simulink model "Validation_test_model_2016"  (Simulink 8.5)
settings: Solver=FixedStepDiscrete  StartTime=0.0  StopTime=10.0  RelTol=1e-3
PreLoadFcn:
  | try, eval([bdroot '_setup']); catch, eval('model_setup', ''); end
InitFcn:
  | try, eval([bdroot '_setup']); catch, eval('model_setup', ''); end
undefined symbols (not defined in the file): a, b, c, d, e, ECU565, f, motohawk_build_version, motohawk_trunc_name, motohawk_vardec_path, sigbuilder_block
libraries: MotoHawk_lib x32, motohawk_annotations_lib x6
Description:
  | Template_of_Final_project
CloseFcn:
  | try, eval([bdroot '_close']); catch, eval('model_close', ''); end
settings Model: MotoHawkBuildVersion=005  MotoHawkBuildStats=struct('TotalFLASH',{0},'TotalEEPROM',{0},'TotalRAM',{0},'AppFLASH',{0},'AppEEPROM',{0},'AppRAM',{0},'HeapRAM',{0},'BuildSuccessCount',{5},'BuildErrorCount',{0})  MotoHawkModelSavedName=Validation_test_model_2016  MotoHawkModelGUID=C2EF9B66-05E6-4C78-8577-5B0F5D47F813  MotoHawkModelOpenTime=2016 3 30 18 59 53.069  MotoHawkModelElapsedTime=96188.182  MotoHawkBuildInfo=struct('model_name',{'Model_in_Template'},'motohawk_version',{'2010a_sp1.49'},'motohawk_component_version',{'0.0.7'},'matlab_version',{'7.10.0'},'build_version',{'004'},'module_type',{'ECU565-128'},'layout_type',{'DEV'},'processor_family',{'PPC'},'processor_type',{'MPC565'},'toolchain_vendor',{'gcc-powerpc-eabi'},'toolchain_version',{'4.4.0'},'component',{0},'archive_file',{'PCM128.a'},'enable_build',{1},'fptype',{0},'flash_size',{1048576},'ee_size',{8192},'ram_size',{36864},'decram_size',{4096},'module_memory_def',{'MPC565_ModMemoryDef_Dev'},'eri_table0_rev',{9},'max_eri_table_size',{65535},'use_debug_vardecs',{1},'use_info_vardecs',{1},'fgnd_base_period_ms',{5},'bgnd_base_period_ms',{50},'root_build_dir',{'C:\MEEM_5750_Final_Project\LeiFeng'},'build_dir',{'C:\MEEM_5750_Final_Project\LeiFeng\Model_in_Template_Build'},'dll_name',{'Model_in__004'},'srz_name',{'Model_in_Template_004'},'fgnd_stack_size',{3072},'fgnd_angle_stack_size',{0},'bgnd_stack_size',{2048},'idle_stack_size',{1024},'irq_stack_size',{1536},'heap_size',{4096},'heap_margin',{409},'install_dll_dir',{'C:\ECUFiles\TDBDLL\'},'install_srz_dir',{'C:\ECUFiles\Programs'},'app_int_stack_size',{1024},'shutdown_stack_size',{1024},'mingw_dir',{'C:\PROGRA~1\Woodward\DEVELO~1\TOOLCH~1\GCC\win32-pe\4_4_0\'},'motohawk_dir',{'C:\PROGRA~1\Woodward\MCS\MotoHawk\2010A_~1.49'},'toolchain_dir',{'C:\Program Files\Woodward\DevelopmentTools\Toolchains\GCC\powerpc-eabi\4_4_0\'},'matlab_root',{'C:\Program Files\matlab2010a'},'model_guid',{'02501405-a1e3-47c9-ad-9c-d2-3e-71-52-84'},'build_guid',{'964a0459-529b-4d6f-81-45-cd-35-ed-ff-d3'},'token_guid',{'FDBF7FB80457F546A307B1464AF6A8B8'})  MotoHawkBuildGUID=964a0459-529b-4d6f-81-45-cd-35-ed-ff-d3  MotoHawkBuildDirectory=C:\Users\Piyush\Desktop\des proj\Validation_test_model_2016_Build  Creator=weiluo  LastModifiedBy=Piyush
settings ConfigSet: Description="This Simulink Configuration Set is preconfigured  for the MotoHawk target \"ECU565-128\"."
settings DataIOCC: SignalLoggingSaveFormat=Dataset
settings OptimizationCC: InlineParams=on  InlineInvariantSignals=on  EnhancedBackFolding=on  ExpressionDepthLimit=128  InitFltsAndDblsToZero=on  NoFixptDivByZeroProtection=on  EfficientFloat2IntCast=on  OptimizeModelRefInitCode=on  LifeSpan=1
settings DebuggingCC: InheritedTsInSrcMsg=none  TasksWithSamePriorityMsg=none  FcnCallInpInsideContextMsg=EnableAllAsError  ModelReferenceIOMismatchMessage=warning  StateNameClashWarn=none
settings HardwareCC: ProdLargestAtomicInteger=Integer  ProdLargestAtomicFloat=Float  ProdEndianess=BigEndian  ProdHWDeviceType=Specified
settings ModelReferenceCC: UpdateModelReferenceTargets=IfOutOfDate  CheckModelReferenceTargetMessage=warning  ModelReferenceNumInstancesAllowed=Single
settings RTWCC: SystemTargetFile=motohawk_ert_rtw.tlc  MakeCommand=make_rtw_motohawk  TemplateMakefile=motohawk_ert_rtw.tmf  Description=MotoHawk(tm) Rapid Prototyping
settings CodeAppCC: IgnoreCustomStorageClasses=off  MaxIdLength=100  CustomSymbolStrType=$N$R$M  CustomSymbolStrField=$H$N$M  InternalIdentifier=Classic
settings STFCustomTargetCC: ERTMultiwordTypeDef=User defined  ERTMultiwordLength=0  IncludeMdlTerminateFcn=off  GeneratePreprocessorConditionals=Disable all  CombineOutputUpdateFcns=on  SuppressErrorStatus=on  ERTCustomFileBanners=on  SupportContinuousTime=off  SupportNonInlinedSFcns=off  MATLABClassNameForMDSCustomization=Simulink.SoftwareTarget.ERTCustomization  GRTInterface=off  SystemTargetFile=motohawk_ert_rtw.tlc
settings ERTTargetCC: ERTMultiwordTypeDef=User defined  ERTMultiwordLength=0  MultiwordLength=2048  ParMdlRefBuildCompliant=off  CompOptLevelCompliant=off  ConcurrentExecutionCompliant=off  IncludeMdlTerminateFcn=off  GeneratePreprocessorConditionals=Disable all  SuppressErrorStatus=on  ERTFirstTimeCompliant=off  ModelStepFunctionPrototypeControlCompliant=off  CPPClassGenCompliant=off  InlinedParameterPlacement=NonHierarchical  ERTCustomFileTemplate=motohawk_file_process.tlc  ConvertIfToSwitch=off  SuppressUnreachableDefaultCases=off
settings CustomProperty: DataType=string  Value=ECU565-128

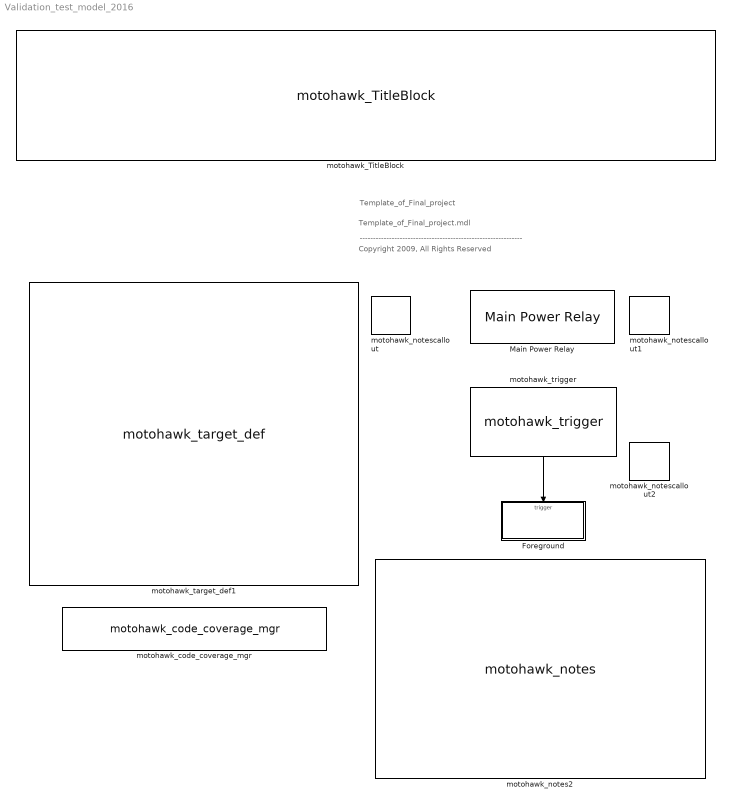
== system Validation_test_model_2016 ==
  note: Template_of_Final_project
  note: Template_of_Final_project.mdl
  note: -------------------------------------------------------------
  note: Copyright 2009, All Rights Reserved
  Foreground : Subsystem  TreatAsAtomicUnit=on
      mask init:
      | SampleTime = 0.005;
      | lbl = sprintf('%d ms', SampleTime * 1000);
      settings: RTWSystemCode=Nonreusable function  RTWFcnNameOpts=Use subsystem name  RTWFileNameOpts=Use function name
      mask Display: disp(lbl);
  Main Power Relay : MotoHawk_lib/Extra Development Blocks/Main Power Relay  on_delay_count=2  off_delay_count=5  ecup_threshold=100  group='System | Main Power Relay'
  motohawk_TitleBlock : motohawk_annotations_lib/motohawk_TitleBlock  BlockType_='Mototron_Title_Block'  ttl="[  strrep(get_param(bdroot, 'Description') , '_', '\\_')  '\\newline\\rm'  'Top-level root of model:  '   strrep(bdroot, '_', '\\_') '.mdl'  ]"  copyright="'THE INFORMATION CONTAINED IN THIS\\newlineDRAWING IS THE SOLE PROPERTY OF\\newlineWOODWARD.  ANY REPRODUCTION IN\\newline PART OR AS A WHOLE WITHOUT THE\\newlineWRITTEN PERMISSION OF WOODWARD\\newline IS PROHIBITED.\\fontsize{16}\\rm\\copyright\\rm\\fontsize{10} 2009'"  address='\fontsize{22}\it\fontname{Arial Black}Woodward \fontname{Arial}\fontsize{10}\newline1000 East Drake Road, Fort Collins, CO, 80525\newlinemcs.woodward.com (866) 588-0494'  image_file='mh.jpg'  pretty_print=on  edit_text=|  edit_as=5
      | [
      | 
      | 
      | 
      | 
      | 
      | strrep(get_param(bdroot, 'Description') , '_', '\_')  '\newline\rm'
      | 
      | 
      | 
      | 
      | 
      | 'Top-level root of model:  '   strrep(bdroot, '_', '\_') '.mdl'
      | 
      | 
      | 
      | 
      | 
      | ]
  motohawk_code_coverage_mgr : MotoHawk_lib/Extra Development Blocks/motohawk_code_coverage_mgr  codegen=Always Generate Code Coverage Code  group='System | Code Coverage'
  motohawk_notes2 : motohawk_annotations_lib/motohawk_notes  BlockType_='Mototron_Notes'  desc="'\\fontname{wingdings 2}u\\fontname{arial}  The existence of a Target Definition block\\newlinesomewhere in the model sets it up as a\\newlineMotoHawk project, capable of being built to a\\newlineMotoTron target module.\\newline\\newline\\fontname{wingdings 2}v\\fontname{arial}  The Main Power Relay block monitors the\\newlinemodule power and controls the Main Power Relay\\newlineIt also performs startup and shutdown procedures\\newlinenecessary for EEPROM storage.  Most designs\\newlineshould contain this block\\newline\\newline\\fontname{wingdings 2}w\\fontname{arial}  All actions must be performed inside of a\\newlinefunction-call subsystem, triggered by a MotoHawk\\newlineentry-point trigger block, in order to be included in the\\newlinegenerated code.\\newline'"  edit_text=|  edit_as=2
      | \fontname{wingdings 2}u\fontname{arial}  The existence of a Target Definition block
      | 
      | 
      | somewhere in the model sets it up as a
      | 
      | 
      | MotoHawk project, capable of being built to a
      | 
      | 
      | Woodward target module.
      | 
      | 
      | 
      | 
      | 
      | \fontname{wingdings 2}v\fontname{arial}  The Main Power Relay block monitors the
      | 
      | 
      | module power and controls the Main Power Relay
      | 
      | 
      | It also performs startup and shutdown procedures
      | 
      | 
      | necessary for EEPROM storage.  Most designs
      | 
      | 
      | should contain this block
      | 
      | 
      | 
      | 
      | 
      | \fontname{wingdings 2}w\fontname{arial}  All actions must be performed inside of a
      | 
      | 
      | function-call subsystem, triggered by a MotoHawk
      | 
      | 
      | entry-point trigger block, in order to be included in the
      | 
      | 
      | generated code.
  motohawk_notescallout : motohawk_annotations_lib/motohawk_notescallout  BlockType_='Mototron_NoteCall'  desc='\bf1'
  motohawk_notescallout1 : motohawk_annotations_lib/motohawk_notescallout  BlockType_='Mototron_NoteCall'  desc='\bf2'
  motohawk_notescallout2 : motohawk_annotations_lib/motohawk_notescallout  BlockType_='Mototron_NoteCall'  desc='\bf3'
  motohawk_target_def1 : MotoHawk_lib/motohawk_target_def  Priority=-65535  target=ECU565-128  layout=DEV  fptype=single (32 bits)  fgnd_stack_size=3*1024  fgnd_angle_stack_size=0  bgnd_stack_size=2*1024  idle_stack_size=1024  irq_stack_size=1536  app_int_stack_size=1024  shutdown_stack_size=1024  heap_size=4*1024  show_margins=off  fgnd_stack_margin=(3*1024) * 0.1  fgnd_angle_stack_margin=0  bgnd_stack_margin=(2*1024) * 0.1  idle_stack_margin=(1024) * 0.1  irq_stack_margin=(1536) * 0.1  app_int_stack_margin=(1024) * 0.1  shutdown_stack_margin=(1024) * 0.1  heap_margin=(4*1024) * 0.1  comp_name=bdroot  comp_img='KVASER_CAN_USB.jpg'  comp_security=No Encryption  comp_build_pass='mhbuild'  comp_sim_pass='mhsim'  comp_multi=off  show_filenames=off  dll_name=motohawk_trunc_name(bdroot, ['_' motohawk_build_version], 13)  srz_name=motohawk_trunc_name(bdroot, ['_' motohawk_build_version], 50)  build_dir='.'  comp_dir='.'
  motohawk_trigger : MotoHawk_lib/Trigger Blocks/motohawk_trigger  Tag=Trigger  Priority=0  trig_name=[]  trigger=FGND_RTI_PERIODIC  priority_order=0  inherited=off  run_disabled=off  override_app_monitor=off  target=ECU565_128
  wires:
  motohawk_trigger/1 -> Foreground/Trigger

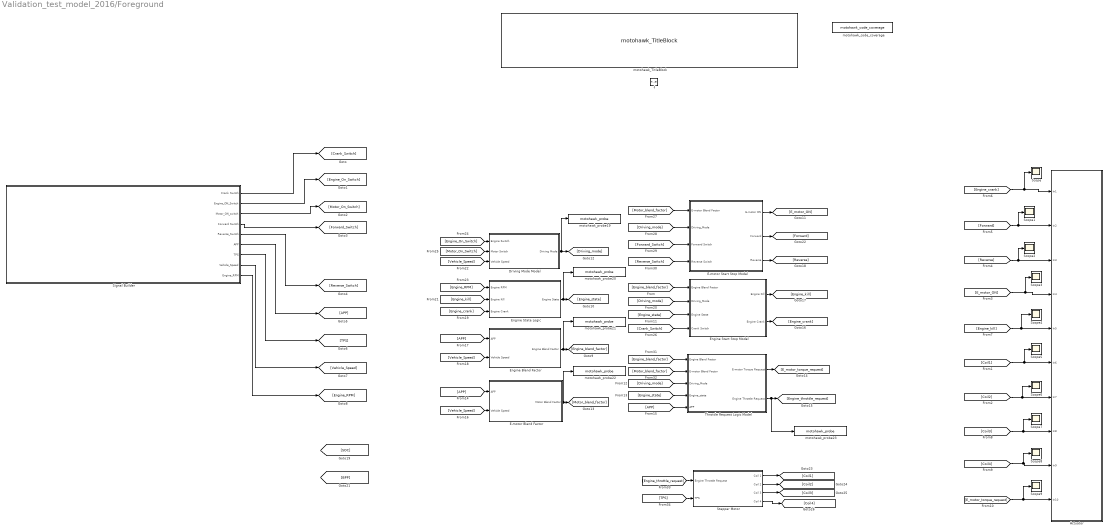
== system Validation_test_model_2016/Foreground ==
  f : TriggerPort  TriggerType=function-call
  Actuator : Subsystem
  Driving Mode Model : Subsystem
  E-motor Blend Factor : Subsystem
  E-motor Start Stop Model : Subsystem
  Engine Blend Factor : Subsystem
  Engine Start Stop Model : Subsystem
  Engine State Logic : Subsystem
  Scope{,1..9} (10 alike) : Scope
      Scope2 settings: TimeRange=10  SaveName=ScopeData2
      Scope3 settings: SaveName=ScopeData3
      Scope4 settings: SaveName=ScopeData4
      Scope5 settings: SaveName=ScopeData5
      Scope6 settings: SaveName=ScopeData6
      Scope7 settings: SaveName=ScopeData7
      Scope8 settings: SaveName=ScopeData8
      Scope9 settings: SaveName=ScopeData9
  Signal Builder : Subsystem  Tag=STV Subsys  LoadFcn=sigbuilder_block('load');  StartFcn=sigbuilder_block('start');  StopFcn=sigbuilder_block('stop');  ClipboardFcn=sigbuilder_block('clipboard');  mask(Sigbuilder block){}
      mask help: Simulink:masks:SigbuilderBlock_MD
      mask init:
      | if ~strcmp(get_param(bdroot(gcbh),'SimulationStatus'),'stopped') tuvar = sigbuilder_block('maskInit'); end
      settings: CopyFcn=sigbuilder_block('copy');  DeleteFcn=sigbuilder_block('delete');  ModelCloseFcn=sigbuilder_block('modelClose');  PreSaveFcn=sigbuilder_block('preSave');  PauseFcn=sigbuilder_block('pause');  ContinueFcn=sigbuilder_block('continue');  NameChangeFcn=sigbuilder_block('namechange');  OpenFcn=sigbuilder_block('open',[437.6 199.2 550.4 400 ]);  CloseFcn=sigbuilder_block('close');
      mask Display: plot(0, 0, 100, 100,[2, 2, 32, 32, 2], [68, 8, 8, 68, 68],[32, 2], [38, 38], [32, 19, 2],[53, 60, 44], [32, 17, 17, 2],[16, 16, 31, 31]);txt = getActiveGroup(gcbh);text(2, 100, txt,'verticalAlignment', 'top');
  Stepper Motor : Subsystem
  Throttle Request Logic Model : Subsystem
  motohawk_TitleBlock : motohawk_annotations_lib/motohawk_TitleBlock  BlockType_='Mototron_Title_Block'  ttl=[strrep(get_param(bdroot, 'Description') , '_', '\_') '\newline\rm' get_param(gcs, 'Name')]  copyright="'THE INFORMATION CONTAINED IN THIS\\newlineDRAWING IS THE SOLE PROPERTY OF\\newlineWOODWARD.  ANY REPRODUCTION IN\\newline PART OR AS A WHOLE WITHOUT THE\\newlineWRITTEN PERMISSION OF WOODWARD\\newline IS PROHIBITED.\\fontsize{16}\\rm\\copyright\\rm\\fontsize{10} 2009'"  address='\fontsize{22}\it\fontname{Arial Black}Woodward \fontname{Arial}\fontsize{10}\newline1000 East Drake Road, Fort Collins, CO, 80525\newlinemcs.woodward.com (866) 588-0494'  image_file='mh.jpg'  pretty_print=on  edit_text=[strrep(get_param(bdroot, 'Description') , '_', '\_') '\newline\rm' get_param(gcs, 'Name')]  edit_as=5
  motohawk_code_coverage : MotoHawk_lib/Extra Development Blocks/motohawk_code_coverage
  motohawk_probe19 : MotoHawk_lib/Calibration & Probing Blocks/motohawk_probe  nam='Driving_Mode'  show_more=off  name_source=Use Parameter  read_level=1  view_as=Number  enum_struct={'Disabled', 'Enabled'}  vector_style=Wide Row  use_help_units=off  help=''  units=''  use_header_enum=off  row_header_enum={}  col_header_enum={}  use_min_max=off  min_val=-inf  max_val=inf  use_precision=off  precision=''  gain=1  offset=0  exp=1  use_mototune_group=off  mototune_group=motohawk_vardec_path(gcb)
  motohawk_probe20 : MotoHawk_lib/Calibration & Probing Blocks/motohawk_probe  nam='Engine_State'  show_more=off  name_source=Use Parameter  read_level=1  view_as=Number  enum_struct={'Disabled', 'Enabled'}  vector_style=Wide Row  use_help_units=off  help=''  units=''  use_header_enum=off  row_header_enum={}  col_header_enum={}  use_min_max=off  min_val=-inf  max_val=inf  use_precision=off  precision=''  gain=1  offset=0  exp=1  use_mototune_group=off  mototune_group=motohawk_vardec_path(gcb)
  motohawk_probe21 : MotoHawk_lib/Calibration & Probing Blocks/motohawk_probe  nam='Engine_Blend_Factor'  show_more=off  name_source=Use Parameter  read_level=1  view_as=Number  enum_struct={'Disabled', 'Enabled'}  vector_style=Wide Row  use_help_units=off  help=''  units=''  use_header_enum=off  row_header_enum={}  col_header_enum={}  use_min_max=off  min_val=-inf  max_val=inf  use_precision=off  precision=''  gain=1  offset=0  exp=1  use_mototune_group=off  mototune_group=motohawk_vardec_path(gcb)
  motohawk_probe22 : MotoHawk_lib/Calibration & Probing Blocks/motohawk_probe  nam='Motor_blend_Factor'  show_more=off  name_source=Use Parameter  read_level=1  view_as=Number  enum_struct={'Disabled', 'Enabled'}  vector_style=Wide Row  use_help_units=off  help=''  units=''  use_header_enum=off  row_header_enum={}  col_header_enum={}  use_min_max=off  min_val=-inf  max_val=inf  use_precision=off  precision=''  gain=1  offset=0  exp=1  use_mototune_group=off  mototune_group=motohawk_vardec_path(gcb)
  motohawk_probe23 : MotoHawk_lib/Calibration & Probing Blocks/motohawk_probe  nam='Engine_Throttle_Request'  show_more=off  name_source=Use Parameter  read_level=1  view_as=Number  enum_struct={'Disabled', 'Enabled'}  vector_style=Wide Row  use_help_units=off  help=''  units=''  use_header_enum=off  row_header_enum={}  col_header_enum={}  use_min_max=off  min_val=-inf  max_val=inf  use_precision=off  precision=''  gain=1  offset=0  exp=1  use_mototune_group=off  mototune_group=motohawk_vardec_path(gcb)
  wires:
  [Forward] -> Scope1/1, Actuator/2(In2)
  [Reverse] -> Scope2/1, Actuator/3(In3)
  [E_motor_ON] -> Scope3/1, Actuator/4(In4)
  [Engine_kill] -> Scope4/1, Actuator/5(In5)
  [Coil1] -> Scope5/1, Actuator/6(In6)
  [Coil2] -> Scope6/1, Actuator/7(In7)
  [Coil3] -> Scope7/1, Actuator/8(In8)
  [Coil4] -> Scope8/1, Actuator/9(In9)
  [E_motor_torque_request] -> Scope9/1, Actuator/10(In10)
  [Engine_blend_factor] -> Engine Start Stop Model/1(Engine Blend Factor)
  Engine State Logic/1(Engine State) -> motohawk_probe20/1, [Engine_state]
  [Engine_state] -> Engine Start Stop Model/3(Engine State)
  Driving Mode Model/1(Driving Mode) -> motohawk_probe19/1, [Driving_mode]
  [Driving_mode] -> Engine Start Stop Model/2(Driving_Mode)
  [Crank_Switch] -> Engine Start Stop Model/4(Crank Switch)
  E-motor Blend Factor/1(Motor Blend Factor) -> motohawk_probe22/1, [Motor_blend_factor]
  [Motor_blend_factor] -> E-motor Start Stop Model/1(E-motor Blend Factor)
  [Driving_mode] -> E-motor Start Stop Model/2(Driving_Mode)
  [Forward_Switch] -> E-motor Start Stop Model/3(Forward Switch)
  [Reverse_Switch] -> E-motor Start Stop Model/4(Reverse Switch)
  [Engine_blend_factor] -> Throttle Request Logic Model/1(Engine Blend Factor)
  [Motor_blend_factor] -> Throttle Request Logic Model/2(E-motor Blend Factor)
  [Driving_mode] -> Throttle Request Logic Model/3(Driving_Mode)
  [Engine_state] -> Throttle Request Logic Model/4(Engine_state)
  [APP] -> E-motor Blend Factor/1(APP)
  [APP] -> Throttle Request Logic Model/5(APP)
  [Vehicle_Speed] -> E-motor Blend Factor/2(Vehicle Speed)
  [APP] -> Engine Blend Factor/1(APP)
  [Vehicle_Speed] -> Engine Blend Factor/2(Vehicle Speed)
  Throttle Request Logic Model/1(E-motor Torque Request) -> [E_motor_torque_request]
  Engine Start Stop Model/2(Engine Crank) -> [Engine_crank]
  Engine Start Stop Model/1(Engine Kill) -> [Engine_kill]
  E-motor Start Stop Model/3(Reverse) -> [Reverse]
  E-motor Start Stop Model/2(Forward) -> [Forward]
  E-motor Start Stop Model/1(E-motor ON) -> [E_motor_ON]
  [Engine_crank] -> Engine State Logic/3(Engine Crank)
  [Engine_kill] -> Engine State Logic/2(Engine Kill)
  [Engine_RPM] -> Engine State Logic/1(Engine RPM)
  [Vehicle_Speed] -> Driving Mode Model/3(Vehicle Speed)
  [Engine_On_Switch] -> Driving Mode Model/1(Engine Switch)
  [Motor_On_Switch] -> Driving Mode Model/2(Motor Switch)
  Engine Blend Factor/1(Engine Blend Factor) -> motohawk_probe21/1, [Engine_blend_factor]
  Throttle Request Logic Model/2(Engine Throttle Request) -> motohawk_probe23/1, [Engine_throttle_request]
  [Engine_throttle_request] -> Stepper Motor/1(Engine Throttle Request)
  [TPS] -> Stepper Motor/2(TPS)
  Stepper Motor/1(Coil 1) -> [Coil1]
  Stepper Motor/2(Coil 2) -> [Coil2]
  Stepper Motor/3(Coil 3) -> [Coil3]
  Stepper Motor/4(Coil 4) -> [Coil4]
  Signal Builder/1(Crank Switch) -> [Crank_Switch]
  Signal Builder/2(Engine_ON_Switch) -> [Engine_On_Switch]
  Signal Builder/3(Motor_ON_switch) -> [Motor_On_Switch]
  Signal Builder/4(Forward Switch) -> [Forward_Switch]
  Signal Builder/5(Reverse_Switch) -> [Reverse_Switch]
  Signal Builder/6(APP) -> [APP]
  [Engine_crank] -> Scope/1, Actuator/1(In1)
  Signal Builder/7(TPS) -> [TPS]
  Signal Builder/8(Vehicle_Speed) -> [Vehicle_Speed]
  Signal Builder/9(Engine_RPM) -> [Engine_RPM]

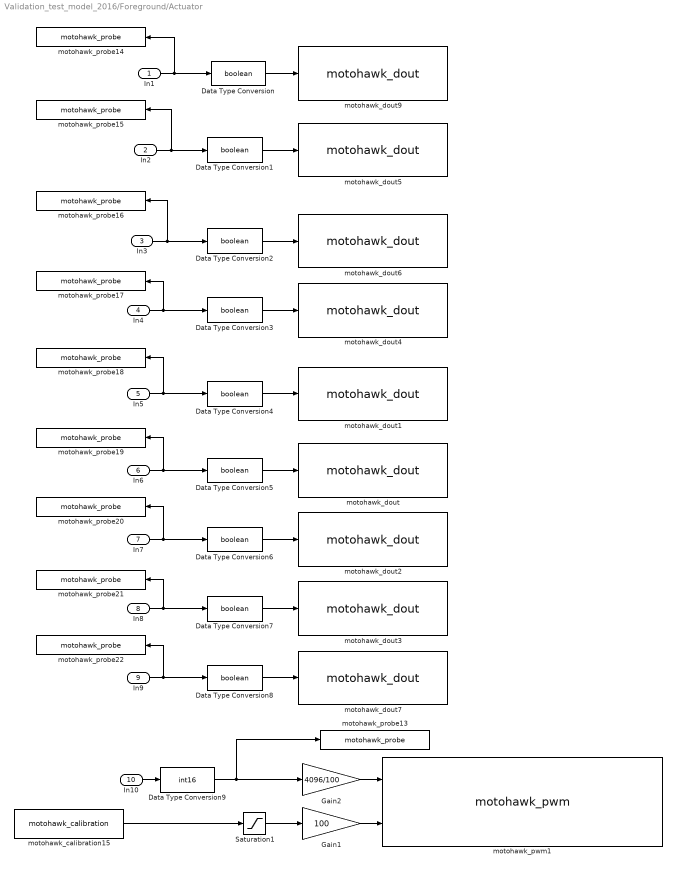
== system Validation_test_model_2016/Foreground/Actuator ==
  In1 : Inport
  In2 : Inport  Port=2
  In3 : Inport  Port=3
  In4 : Inport  Port=4
  In5 : Inport  Port=5
  In6 : Inport  Port=6
  In7 : Inport  Port=7
  In8 : Inport  Port=8
  In9 : Inport  Port=9
  In10 : Inport  Port=10
  Data Type Conversion{,1..8} (9 alike) : DataTypeConversion  OutDataTypeStr=boolean
  Data Type Conversion9 : DataTypeConversion  OutDataTypeStr=int16
  Gain1 : Gain  Gain=100  OutDataTypeStr=Inherit: Inherit via back propagation
  Gain2 : Gain  Gain=4096/100  OutDataTypeStr=Inherit: Inherit via back propagation
  Saturation1 : Saturate  UpperLimit=10000  LowerLimit=0
  motohawk_calibration15 : MotoHawk_lib/Calibration & Probing Blocks/motohawk_calibration  nam='Throttle_Frequency'  val=10000  storage=Calibration  show_more=on  name_source=Use Parameter  data_type=Inherit via back propagation  read_level=1  write_level=1  ovr_cals=on  view_as=Number  enum_struct={'Disabled', 'Enabled'}  vector_style=Wide Row  use_help_units=off  help=''  units=''  use_header_enum=off  row_header_enum={}  col_header_enum={}  use_min_max=off  min_val=-inf  max_val=inf  use_precision=off  precision=''  gain=1  offset=0  exp=1  use_mototune_group=off  mototune_group=motohawk_vardec_path(gcb)  data_stores=motohawk_sfun_calibration_data_stores
  motohawk_dout : MotoHawk_lib/Digital I//O Blocks/motohawk_dout  resource_name=[]  text_resource=LSD5  target=ECU565-128  use_diag=off  use_vardec=off  nam='DOUT'  read_level=1  write_level=1  group='System | I/O Pins | Outputs Config'
  motohawk_dout1 : MotoHawk_lib/Digital I//O Blocks/motohawk_dout  resource_name=[]  text_resource=LSD9  target=ECU565-128  use_diag=off  use_vardec=off  nam='DOUT'  read_level=1  write_level=1  group='System | I/O Pins | Outputs Config'
  motohawk_dout2 : MotoHawk_lib/Digital I//O Blocks/motohawk_dout  resource_name=[]  text_resource=LSD6  target=ECU565-128  use_diag=off  use_vardec=off  nam='DOUT'  read_level=1  write_level=1  group='System | I/O Pins | Outputs Config'
  motohawk_dout3 : MotoHawk_lib/Digital I//O Blocks/motohawk_dout  resource_name=[]  text_resource=LSD7  target=ECU565-128  use_diag=off  use_vardec=off  nam='DOUT'  read_level=1  write_level=1  group='System | I/O Pins | Outputs Config'
  motohawk_dout4 : MotoHawk_lib/Digital I//O Blocks/motohawk_dout  resource_name=[]  text_resource=LSD4  target=ECU565-128  use_diag=off  use_vardec=off  nam='DOUT'  read_level=1  write_level=1  group='System | I/O Pins | Outputs Config'
  motohawk_dout5 : MotoHawk_lib/Digital I//O Blocks/motohawk_dout  resource_name=[]  text_resource=LSD2  target=ECU565-128  use_diag=off  use_vardec=off  nam='DOUT'  read_level=1  write_level=1  group='System | I/O Pins | Outputs Config'
  motohawk_dout6 : MotoHawk_lib/Digital I//O Blocks/motohawk_dout  resource_name=[]  text_resource=LSD3  target=ECU565-128  use_diag=off  use_vardec=off  nam='DOUT'  read_level=1  write_level=1  group='System | I/O Pins | Outputs Config'
  motohawk_dout7 : MotoHawk_lib/Digital I//O Blocks/motohawk_dout  resource_name=[]  text_resource=LSD8  target=ECU565-128  use_diag=off  use_vardec=off  nam='DOUT'  read_level=1  write_level=1  group='System | I/O Pins | Outputs Config'
  motohawk_dout9 : MotoHawk_lib/Digital I//O Blocks/motohawk_dout  resource_name=[]  text_resource=LSD1  target=ECU565-128  use_diag=off  use_vardec=off  nam='DOUT'  read_level=1  write_level=1  group='System | I/O Pins | Outputs Config'
  motohawk_probe13 : MotoHawk_lib/Calibration & Probing Blocks/motohawk_probe  nam='Emotor_Throttle_Request'  show_more=off  name_source=Use Parameter  read_level=1  view_as=Number  enum_struct={'Disabled', 'Enabled'}  vector_style=Wide Row  use_help_units=off  help=''  units=''  use_header_enum=off  row_header_enum={}  col_header_enum={}  use_min_max=off  min_val=-inf  max_val=inf  use_precision=off  precision=''  gain=1  offset=0  exp=1  use_mototune_group=off  mototune_group=motohawk_vardec_path(gcb)
  motohawk_probe14 : MotoHawk_lib/Calibration & Probing Blocks/motohawk_probe  nam='Engine_Crank'  show_more=off  name_source=Use Parameter  read_level=1  view_as=Number  enum_struct={'Disabled', 'Enabled'}  vector_style=Wide Row  use_help_units=off  help=''  units=''  use_header_enum=off  row_header_enum={}  col_header_enum={}  use_min_max=off  min_val=-inf  max_val=inf  use_precision=off  precision=''  gain=1  offset=0  exp=1  use_mototune_group=off  mototune_group=motohawk_vardec_path(gcb)
  motohawk_probe15 : MotoHawk_lib/Calibration & Probing Blocks/motohawk_probe  nam='Foward'  show_more=off  name_source=Use Parameter  read_level=1  view_as=Number  enum_struct={'Disabled', 'Enabled'}  vector_style=Wide Row  use_help_units=off  help=''  units=''  use_header_enum=off  row_header_enum={}  col_header_enum={}  use_min_max=off  min_val=-inf  max_val=inf  use_precision=off  precision=''  gain=1  offset=0  exp=1  use_mototune_group=off  mototune_group=motohawk_vardec_path(gcb)
  motohawk_probe16 : MotoHawk_lib/Calibration & Probing Blocks/motohawk_probe  nam='Reverse'  show_more=off  name_source=Use Parameter  read_level=1  view_as=Number  enum_struct={'Disabled', 'Enabled'}  vector_style=Wide Row  use_help_units=off  help=''  units=''  use_header_enum=off  row_header_enum={}  col_header_enum={}  use_min_max=off  min_val=-inf  max_val=inf  use_precision=off  precision=''  gain=1  offset=0  exp=1  use_mototune_group=off  mototune_group=motohawk_vardec_path(gcb)
  motohawk_probe17 : MotoHawk_lib/Calibration & Probing Blocks/motohawk_probe  nam='E_Motor_On'  show_more=off  name_source=Use Parameter  read_level=1  view_as=Number  enum_struct={'Disabled', 'Enabled'}  vector_style=Wide Row  use_help_units=off  help=''  units=''  use_header_enum=off  row_header_enum={}  col_header_enum={}  use_min_max=off  min_val=-inf  max_val=inf  use_precision=off  precision=''  gain=1  offset=0  exp=1  use_mototune_group=off  mototune_group=motohawk_vardec_path(gcb)
  motohawk_probe18 : MotoHawk_lib/Calibration & Probing Blocks/motohawk_probe  nam='Engine_Kill'  show_more=off  name_source=Use Parameter  read_level=1  view_as=Number  enum_struct={'Disabled', 'Enabled'}  vector_style=Wide Row  use_help_units=off  help=''  units=''  use_header_enum=off  row_header_enum={}  col_header_enum={}  use_min_max=off  min_val=-inf  max_val=inf  use_precision=off  precision=''  gain=1  offset=0  exp=1  use_mototune_group=off  mototune_group=motohawk_vardec_path(gcb)
  motohawk_probe19 : MotoHawk_lib/Calibration & Probing Blocks/motohawk_probe  nam='Coil_1'  show_more=off  name_source=Use Parameter  read_level=1  view_as=Number  enum_struct={'Disabled', 'Enabled'}  vector_style=Wide Row  use_help_units=off  help=''  units=''  use_header_enum=off  row_header_enum={}  col_header_enum={}  use_min_max=off  min_val=-inf  max_val=inf  use_precision=off  precision=''  gain=1  offset=0  exp=1  use_mototune_group=off  mototune_group=motohawk_vardec_path(gcb)
  motohawk_probe20 : MotoHawk_lib/Calibration & Probing Blocks/motohawk_probe  nam='Coil_2'  show_more=off  name_source=Use Parameter  read_level=1  view_as=Number  enum_struct={'Disabled', 'Enabled'}  vector_style=Wide Row  use_help_units=off  help=''  units=''  use_header_enum=off  row_header_enum={}  col_header_enum={}  use_min_max=off  min_val=-inf  max_val=inf  use_precision=off  precision=''  gain=1  offset=0  exp=1  use_mototune_group=off  mototune_group=motohawk_vardec_path(gcb)
  motohawk_probe21 : MotoHawk_lib/Calibration & Probing Blocks/motohawk_probe  nam='Coil_3'  show_more=off  name_source=Use Parameter  read_level=1  view_as=Number  enum_struct={'Disabled', 'Enabled'}  vector_style=Wide Row  use_help_units=off  help=''  units=''  use_header_enum=off  row_header_enum={}  col_header_enum={}  use_min_max=off  min_val=-inf  max_val=inf  use_precision=off  precision=''  gain=1  offset=0  exp=1  use_mototune_group=off  mototune_group=motohawk_vardec_path(gcb)
  motohawk_probe22 : MotoHawk_lib/Calibration & Probing Blocks/motohawk_probe  nam='Coil_4'  show_more=off  name_source=Use Parameter  read_level=1  view_as=Number  enum_struct={'Disabled', 'Enabled'}  vector_style=Wide Row  use_help_units=off  help=''  units=''  use_header_enum=off  row_header_enum={}  col_header_enum={}  use_min_max=off  min_val=-inf  max_val=inf  use_precision=off  precision=''  gain=1  offset=0  exp=1  use_mototune_group=off  mototune_group=motohawk_vardec_path(gcb)
  motohawk_pwm1 : MotoHawk_lib/Analog I//O Blocks/motohawk_pwm  res_name='Emotor_Throttle'  text_resource=EST 1  target=ECU565-128  freq_mode=-1  min_freq=2  use_max_freq=off  max_freq=42949672.96  use_enable=off  use_brake=off  output_current=off  output_fault_status=off  use_child=off  use_vardec=off  nam='PWM'  read_level=1  write_level=1  group='System | I/O Pins | Outputs Config'
  wires:
  Data Type Conversion9/1 -> motohawk_probe13/1, Gain2/1
  Data Type Conversion8/1 -> motohawk_dout7/1
  Data Type Conversion7/1 -> motohawk_dout3/1
  Data Type Conversion6/1 -> motohawk_dout2/1
  Data Type Conversion5/1 -> motohawk_dout/1
  Data Type Conversion4/1 -> motohawk_dout1/1
  Data Type Conversion3/1 -> motohawk_dout4/1
  Data Type Conversion2/1 -> motohawk_dout6/1
  Data Type Conversion1/1 -> motohawk_dout5/1
  Data Type Conversion/1 -> motohawk_dout9/1
  In9/1 -> Data Type Conversion8/1, motohawk_probe22/1
  In8/1 -> Data Type Conversion7/1, motohawk_probe21/1
  In7/1 -> Data Type Conversion6/1, motohawk_probe20/1
  In6/1 -> Data Type Conversion5/1, motohawk_probe19/1
  Saturation1/1 -> Gain1/1
  Gain2/1 -> motohawk_pwm1/1
  Gain1/1 -> motohawk_pwm1/2
  motohawk_calibration15/1 -> Saturation1/1
  In2/1 -> Data Type Conversion1/1, motohawk_probe15/1
  In5/1 -> Data Type Conversion4/1, motohawk_probe18/1
  In1/1 -> Data Type Conversion/1, motohawk_probe14/1
  In3/1 -> Data Type Conversion2/1, motohawk_probe16/1
  In4/1 -> Data Type Conversion3/1, motohawk_probe17/1
  In10/1 -> Data Type Conversion9/1

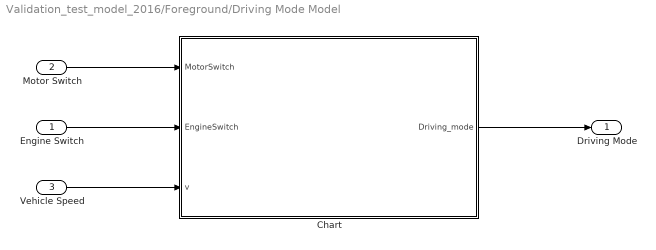
== system Validation_test_model_2016/Foreground/Driving Mode Model ==
  Engine Switch : Inport
  Motor Switch : Inport  Port=2
  Vehicle Speed : Inport  Port=3
  Chart : Stateflow chart  TreatAsAtomicUnit=on
  Driving Mode : Outport
  wires:
  Motor Switch/1 -> Chart/1(MotorSwitch)
  Engine Switch/1 -> Chart/2(EngineSwitch)
  Vehicle Speed/1 -> Chart/3(v)
  Chart/1(Driving_mode) -> Driving Mode/1

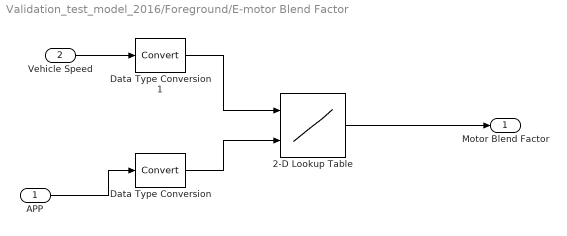
== system Validation_test_model_2016/Foreground/E-motor Blend Factor ==
  APP : Inport
  Vehicle Speed : Inport  Port=2
  2-D Lookup Table : Lookup_n-D  BreakpointsForDimension1=a  BreakpointsForDimension2=b  Table=c  InternalRulePriority=Speed  RndMeth=Simplest  InputSameDT=on
  Data Type Conversion : DataTypeConversion
  Data Type Conversion1 : DataTypeConversion
  Motor Blend Factor : Outport
  wires:
  Vehicle Speed/1 -> Data Type Conversion1/1
  APP/1 -> Data Type Conversion/1
  2-D Lookup Table/1 -> Motor Blend Factor/1
  Data Type Conversion/1 -> 2-D Lookup Table/2
  Data Type Conversion1/1 -> 2-D Lookup Table/1

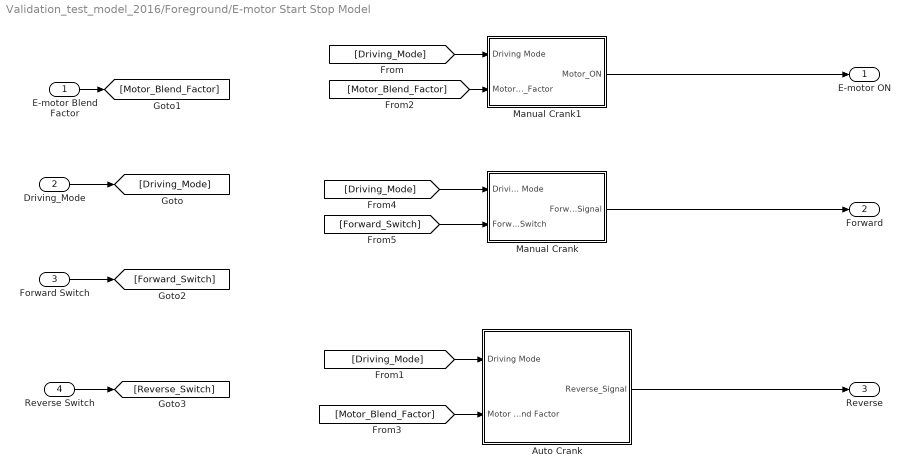
== system Validation_test_model_2016/Foreground/E-motor Start Stop Model ==
  E-motor Blend Factor : Inport
  Driving_Mode : Inport  Port=2
  Forward Switch : Inport  Port=3
  Reverse Switch : Inport  Port=4
  Auto Crank : Subsystem
  Manual Crank : Subsystem
  Manual Crank1 : Subsystem
  E-motor ON : Outport
  Forward : Outport  Port=2
  Reverse : Outport  Port=3
  wires:
  [Forward_Switch] -> Manual Crank/2(Forward Switch)
  Manual Crank1/1(Motor_ON) -> E-motor ON/1
  [Driving_Mode] -> Manual Crank1/1(Driving Mode)
  [Driving_Mode] -> Auto Crank/1(Driving Mode)
  [Motor_Blend_Factor] -> Manual Crank1/2(Motor_Blend_Factor)
  [Motor_Blend_Factor] -> Auto Crank/2(Motor Blend Factor)
  [Driving_Mode] -> Manual Crank/1(Driving Mode)
  E-motor Blend Factor/1 -> [Motor_Blend_Factor]
  Driving_Mode/1 -> [Driving_Mode]
  Forward Switch/1 -> [Forward_Switch]
  Reverse Switch/1 -> [Reverse_Switch]
  Auto Crank/1(Reverse_Signal) -> Reverse/1
  Manual Crank/1(Forward_Signal) -> Forward/1

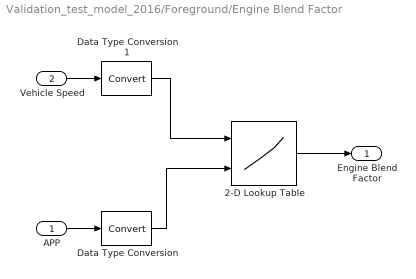
== system Validation_test_model_2016/Foreground/Engine Blend Factor ==
  APP : Inport
  Vehicle Speed : Inport  Port=2
  2-D Lookup Table : Lookup_n-D  BreakpointsForDimension1=d  BreakpointsForDimension2=e  Table=f  InternalRulePriority=Speed  RndMeth=Simplest  InputSameDT=on
  Data Type Conversion : DataTypeConversion
  Data Type Conversion1 : DataTypeConversion
  Engine Blend Factor : Outport
  wires:
  2-D Lookup Table/1 -> Engine Blend Factor/1
  APP/1 -> Data Type Conversion/1
  Vehicle Speed/1 -> Data Type Conversion1/1
  Data Type Conversion/1 -> 2-D Lookup Table/2
  Data Type Conversion1/1 -> 2-D Lookup Table/1

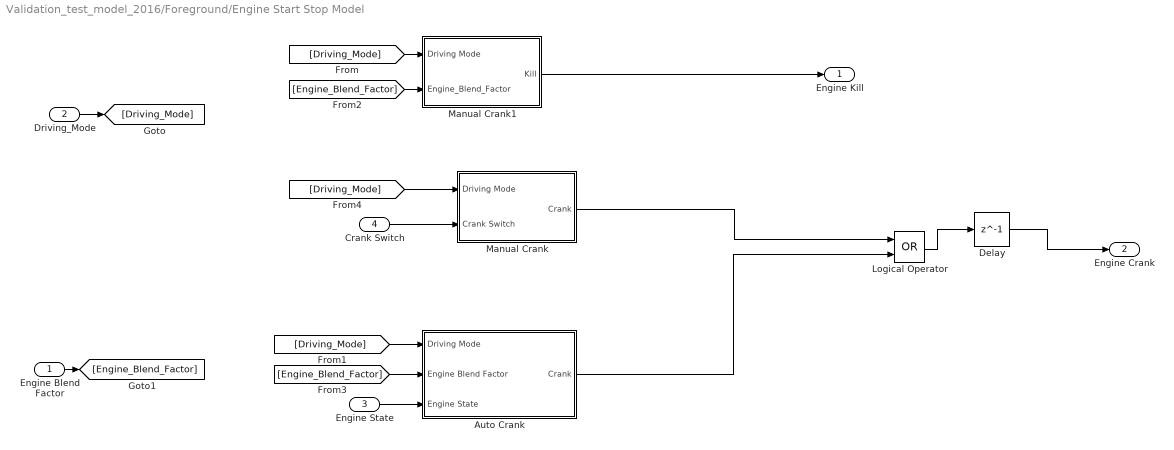
== system Validation_test_model_2016/Foreground/Engine Start Stop Model ==
  Engine Blend Factor : Inport
  Driving_Mode : Inport  Port=2
  Engine State : Inport  Port=3
  Crank Switch : Inport  Port=4
  Auto Crank : Subsystem
  Delay : Delay  DelayLength=1  InitialCondition=0
  Logical Operator : Logic  Operator=OR  AllPortsSameDT=off  OutDataTypeStr=boolean
  Manual Crank : Subsystem
  Manual Crank1 : Subsystem
  Engine Kill : Outport
  Engine Crank : Outport  Port=2
  wires:
  Logical Operator/1 -> Delay/1
  Crank Switch/1 -> Manual Crank/2(Crank Switch)
  Engine State/1 -> Auto Crank/3(Engine State)
  Manual Crank1/1(Kill) -> Engine Kill/1
  Driving_Mode/1 -> [Driving_Mode]
  Engine Blend Factor/1 -> [Engine_Blend_Factor]
  [Driving_Mode] -> Manual Crank1/1(Driving Mode)
  [Driving_Mode] -> Auto Crank/1(Driving Mode)
  [Engine_Blend_Factor] -> Manual Crank1/2(Engine_Blend_Factor)
  [Engine_Blend_Factor] -> Auto Crank/2(Engine Blend Factor)
  [Driving_Mode] -> Manual Crank/1(Driving Mode)
  Auto Crank/1(Crank) -> Logical Operator/2
  Manual Crank/1(Crank) -> Logical Operator/1
  Delay/1 -> Engine Crank/1

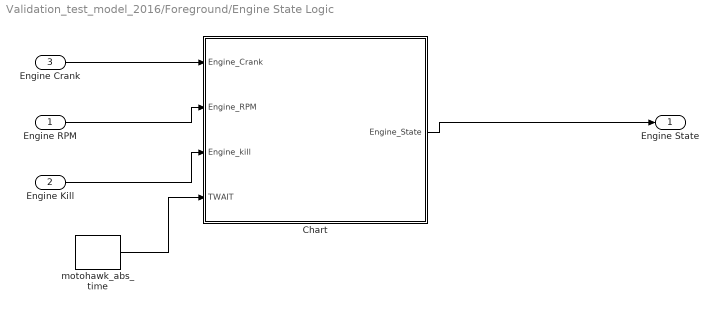
== system Validation_test_model_2016/Foreground/Engine State Logic ==
  Engine RPM : Inport
  Engine Kill : Inport  Port=2
  Engine Crank : Inport  Port=3
  Chart : Stateflow chart  TreatAsAtomicUnit=on
  motohawk_abs_time : MotoHawk_lib/Extra Development Blocks/motohawk_abs_time  mode=Seconds (double)  width=64 bit
  Engine State : Outport
  wires:
  Engine Crank/1 -> Chart/1(Engine_Crank)
  Engine Kill/1 -> Chart/3(Engine_kill)
  Engine RPM/1 -> Chart/2(Engine_RPM)
  Chart/1(Engine_State) -> Engine State/1
  motohawk_abs_time/1 -> Chart/4(TWAIT)

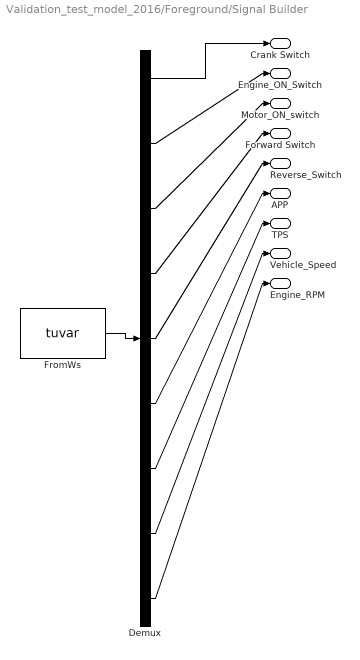
== system Validation_test_model_2016/Foreground/Signal Builder ==
  Demux : Demux  Tag=STV Demux  Outputs=9
  FromWs : FromWorkspace  Tag=STV FromWs  VariableName=tuvar  SigBuilderData=DataTag0  VnvData=DataTag1
      SigBuilderData=|
      | common.afterFinalStr = 'Extrapolate'
      | common.sampleTime = '-1'
      | dataSet.timeRange = [0 10]
      | dataSet.name = 'Group 1'
      | sbobj.Groups.Name = 'Group 1'
      | sbobj.Groups.Signals(1).Name = 'Crank Switch'
      | sbobj.Groups.Signals(1).XData = [0 4 6 10]
      | sbobj.Groups.Signals(1).YData = [0 0 0 0]
      | sbobj.Groups.Signals(2).Name = 'Engine_ON_Switch'
      | sbobj.Groups.Signals(2).XData = [0 10]
      | sbobj.Groups.Signals(2).YData = [1 1]
      | sbobj.Groups.Signals(3).Name = 'Motor_ON_switch'
      | sbobj.Groups.Signals(3).XData = [0 10]
      | sbobj.Groups.Signals(3).YData = [1 1]
      | sbobj.Groups.Signals(4).Name = 'Forward Switch'
      | sbobj.Groups.Signals(4).XData = [0 10]
      | sbobj.Groups.Signals(4).YData = [1 1]
      | sbobj.Groups.Signals(5).Name = 'Reverse_Switch'
      | sbobj.Groups.Signals(5).XData = [0 10]
      | sbobj.Groups.Signals(5).YData = [0 0.7]
      | sbobj.Groups.Signals(6).Name = 'APP'
      | sbobj.Groups.Signals(6).XData = [0 10]
      | sbobj.Groups.Signals(6).YData = [0 0.8]
      | sbobj.Groups.Signals(7).Name = 'TPS'
      | sbobj.Groups.Signals(7).XData = [0 1 10]
      | sbobj.Groups.Signals(7).YData = [0 2000 2000]
      | sbobj.Groups.Signals(8).Name = 'Vehicle_Speed'
      | sbobj.Groups.Signals(8).XData = [0 10]
      | sbobj.Groups.Signals(8).YData = [0 0]
      | sbobj.Groups.Signals(9).Name = 'Engine_RPM'
      | sbobj.Groups.Signals(9).XData = [0 10]
      | sbobj.Groups.Signals(9).YData = [0 0]
  Crank Switch : Outport  Tag=STV Outport
  Engine_ON_Switch : Outport  Tag=STV Outport  Port=2
  Motor_ON_switch : Outport  Tag=STV Outport  Port=3
  Forward Switch : Outport  Tag=STV Outport  Port=4
  Reverse_Switch : Outport  Tag=STV Outport  Port=5
  APP : Outport  Tag=STV Outport  Port=6
  TPS : Outport  Tag=STV Outport  Port=7
  Vehicle_Speed : Outport  Tag=STV Outport  Port=8
  Engine_RPM : Outport  Tag=STV Outport  Port=9
  wires:
  Demux/1 -> Crank Switch/1
  FromWs/1 -> Demux/1
  Demux/2 -> Engine_ON_Switch/1
  Demux/3 -> Motor_ON_switch/1
  Demux/4 -> Forward Switch/1
  Demux/5 -> Reverse_Switch/1
  Demux/6 -> APP/1
  Demux/7 -> TPS/1
  Demux/8 -> Vehicle_Speed/1
  Demux/9 -> Engine_RPM/1

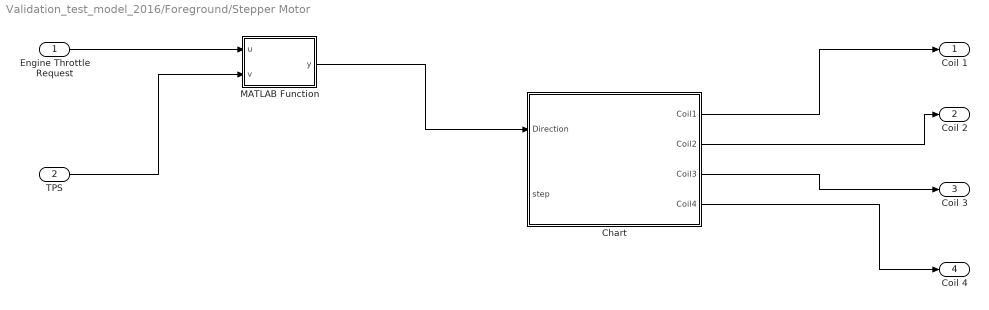
== system Validation_test_model_2016/Foreground/Stepper Motor ==
  Engine Throttle Request : Inport
  TPS : Inport  Port=2
  Chart : Stateflow chart  TreatAsAtomicUnit=on
  MATLAB Function : MATLAB Function  TreatAsAtomicUnit=on
  Coil 1 : Outport
  Coil 2 : Outport  Port=2
  Coil 3 : Outport  Port=3
  Coil 4 : Outport  Port=4
  wires:
  Engine Throttle Request/1 -> MATLAB Function/1(u)
  TPS/1 -> MATLAB Function/2(v)
  MATLAB Function/1(y) -> Chart/1(Direction)
  Chart/1(Coil1) -> Coil 1/1
  Chart/2(Coil2) -> Coil 2/1
  Chart/3(Coil3) -> Coil 3/1
  Chart/4(Coil4) -> Coil 4/1

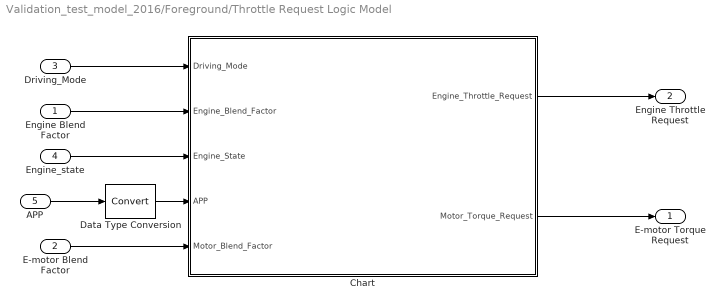
== system Validation_test_model_2016/Foreground/Throttle Request Logic Model ==
  Engine Blend Factor : Inport
  E-motor Blend Factor : Inport  Port=2
  Driving_Mode : Inport  Port=3
  Engine_state : Inport  Port=4
  APP : Inport  Port=5
  Chart : Stateflow chart  TreatAsAtomicUnit=on
  Data Type Conversion : DataTypeConversion
  E-motor Torque Request : Outport
  Engine Throttle Request : Outport  Port=2
  wires:
  Engine Blend Factor/1 -> Chart/2(Engine_Blend_Factor)
  E-motor Blend Factor/1 -> Chart/5(Motor_Blend_Factor)
  APP/1 -> Data Type Conversion/1
  Engine_state/1 -> Chart/3(Engine_State)
  Driving_Mode/1 -> Chart/1(Driving_Mode)
  Chart/2(Motor_Torque_Request) -> E-motor Torque Request/1
  Chart/1(Engine_Throttle_Request) -> Engine Throttle Request/1
  Data Type Conversion/1 -> Chart/4(APP)

== system Validation_test_model_2016/Foreground/E-motor Start Stop Model/Auto Crank ==
  Driving Mode : Inport
  Motor Blend Factor : Inport  Port=2
  Chart2 : Stateflow chart  TreatAsAtomicUnit=on
  Reverse_Signal : Outport
  wires:
  Chart2/1(Reverse) -> Reverse_Signal/1
  Driving Mode/1 -> Chart2/1(Driving_Mode)
  Motor Blend Factor/1 -> Chart2/2(Reverse_switch)

== system Validation_test_model_2016/Foreground/E-motor Start Stop Model/Manual Crank ==
  Driving Mode : Inport
  Forward Switch : Inport  Port=2
  Chart1 : Stateflow chart  TreatAsAtomicUnit=on
  Forward_Signal : Outport
  wires:
  Chart1/1(Forward) -> Forward_Signal/1
  Driving Mode/1 -> Chart1/1(Driving_Mode)
  Forward Switch/1 -> Chart1/2(Forward_switch)

== system Validation_test_model_2016/Foreground/E-motor Start Stop Model/Manual Crank1 ==
  Driving Mode : Inport
  Motor_Blend_Factor : Inport  Port=2
  Chart1 : Stateflow chart  TreatAsAtomicUnit=on
  Motor_ON : Outport
  wires:
  Driving Mode/1 -> Chart1/1(Driving_Mode)
  Motor_Blend_Factor/1 -> Chart1/2(Motor_Blend_Factor)
  Chart1/1(Motor_on) -> Motor_ON/1

== system Validation_test_model_2016/Foreground/Engine Start Stop Model/Auto Crank ==
  Driving Mode : Inport
  Engine Blend Factor : Inport  Port=2
  Engine State : Inport  Port=3
  Chart2 : Stateflow chart  TreatAsAtomicUnit=on
  Crank : Outport
  wires:
  Chart2/1(Automatic_crank) -> Crank/1
  Engine State/1 -> Chart2/3(Engine_State)
  Engine Blend Factor/1 -> Chart2/2(Engine_Blend_Factor)
  Driving Mode/1 -> Chart2/1(Driving_Mode)

== system Validation_test_model_2016/Foreground/Engine Start Stop Model/Manual Crank ==
  Driving Mode : Inport
  Crank Switch : Inport  Port=2
  Chart1 : Stateflow chart  TreatAsAtomicUnit=on
  Crank : Outport
  wires:
  Driving Mode/1 -> Chart1/1(Driving_Mode)
  Crank Switch/1 -> Chart1/2(Crank_Switch)
  Chart1/1(Manual_crank) -> Crank/1

== system Validation_test_model_2016/Foreground/Engine Start Stop Model/Manual Crank1 ==
  Driving Mode : Inport
  Engine_Blend_Factor : Inport  Port=2
  Chart1 : Stateflow chart  TreatAsAtomicUnit=on
  Kill : Outport
  wires:
  Engine_Blend_Factor/1 -> Chart1/2(Engine_Blend_Factor)
  Driving Mode/1 -> Chart1/1(Driving_Mode)
  Chart1/1(Engine_Kill) -> Kill/1

== stateflow chart Foreground/Engine State Logic/Chart ==
  state EngineCrank
    en: Time_stamp = TWAIT;
    during:Engine_State=2;
  state EngineOff
    during:Engine_State=1;
  state EngineStartFailSate
    during:Engine_State=5;
  state EngineOn
    en: Time_stamp = TWAIT;
    during:Engine_State=4;
  state EngineWarm_up
    en: Time_stamp = TWAIT;
    during: Engine_State=3;
  (default) -> EngineOff
  EngineOff -> EngineCrank : [Engine_Crank==1]
  EngineCrank -> EngineStartFailSate [order 2] : [Engine_RPM<=800&&TWAIT>Time_stamp+1]
  EngineCrank -> EngineWarm_up [order 1] : [Engine_RPM>800&&TWAIT>Time_stamp+0.6]
  EngineStartFailSate -> EngineOff
  EngineOn -> EngineOff : [Engine_RPM<50||Engine_kill==1]
  EngineWarm_up -> EngineStartFailSate [order 2] : [Engine_RPM<500 && TWAIT>Time_stamp+1]
  EngineWarm_up -> EngineOn [order 1] : [Engine_RPM>=500&&TWAIT>Time_stamp+1]
  data: Engine_Crank input double; Engine_RPM input double; Engine_kill input double; Engine_State output double; TWAIT input double; Time_stamp local double

== stateflow chart Foreground/E-motor Start Stop Model/Auto Crank/Chart2 ==
  state REVERSE_ON
    during: Reverse=1;
  state REVERSE_OFF
    during: Reverse=0;
  REVERSE_ON -> REVERSE_OFF : [Driving_Mode==2||Driving_Mode==3]
  REVERSE_OFF -> REVERSE_ON : [Driving_Mode==1&&Reverse_switch==1]
  (default) -> REVERSE_OFF
  data: Driving_Mode input double; Reverse_switch input double; Reverse output double

== stateflow chart Foreground/Driving Mode Model/Chart ==
  state Electric_solo_mode
    during:Driving_mode=1;
  state Blending_mode
    during:Driving_mode=2;
  state Engine_Solo_mode
    during: Driving_mode=3;
  (junction 41) -> Electric_solo_mode [order 2] : [MotorSwitch==1&&EngineSwitch==0&&v<1]
  Electric_solo_mode -> (junction 41) : [MotorSwitch==0&&v<1]
  (default) -> Blending_mode
  (junction 41) -> Blending_mode [order 3] : [EngineSwitch==0&&MotorSwitch==0&&v<1]
  Blending_mode -> (junction 41) : [EngineSwitch==0||MotorSwitch==0&&v<1]
  Engine_Solo_mode -> (junction 41) : [EngineSwitch==0&&v<1]
  (junction 41) -> Engine_Solo_mode [order 1] : [EngineSwitch==1&&MotorSwitch==0&&v<1]
  data: MotorSwitch input double; EngineSwitch input double; v input double; Driving_mode output double

== stateflow chart Foreground/Throttle Request Logic Model/Chart ==
  state BlendingMode
    state State1
      during: Engine_Throttle_Request=7.5;
      during:Motor_Torque_Request=APP*Motor_Blend_Factor;
    state State2
      during: Engine_Throttle_Request=(APP*Engine_Blend_Factor);
      during: Motor_Torque_Request=APP*Motor_Blend_Factor;
    State2 -> State1 : [Engine_State==2||Engine_State==3]
    State1 -> State2 : [Engine_State==1||Engine_State==4||Engine_State==5]
    (default) -> State2
  state ElectricSoloMode
    during: Engine_Throttle_Request=0;
    during: Motor_Torque_Request=APP;
  state EngineSoloMode
    during:Engine_Throttle_Request=APP;
    during: Motor_Torque_Request = 0;
  (default) -> ElectricSoloMode
  ElectricSoloMode -> (junction 66) : [Driving_Mode==2||Driving_Mode==3]
  (junction 66) -> ElectricSoloMode [order 1] : [Driving_Mode==1]
  (junction 66) -> BlendingMode [order 2] : [Driving_Mode==2]
  (junction 66) -> EngineSoloMode [order 3] : [Driving_Mode==3]
  BlendingMode -> (junction 66) : [Driving_Mode==2||Driving_Mode==1]
  EngineSoloMode -> (junction 66) : [Driving_Mode==2||Driving_Mode==1]
  data: Driving_Mode input double; Engine_Blend_Factor input double; Engine_State input double; APP input double; Motor_Blend_Factor input double; Engine_Throttle_Request output double; Motor_Torque_Request output double

== stateflow chart Foreground/E-motor Start Stop Model/Manual Crank/Chart1 ==
  state FORWARD_ON
    during: Forward=1;
  state FORWARD_OFF
    during: Forward=0;
  FORWARD_ON -> FORWARD_OFF : [Driving_Mode==3]
  FORWARD_OFF -> FORWARD_ON [order 1] : [Driving_Mode==2]
  FORWARD_OFF -> FORWARD_ON [order 2] : [Driving_Mode==1&&Forward_switch==1]
  (default) -> FORWARD_OFF
  data: Driving_Mode input double; Forward_switch input double; Forward output double

== stateflow chart Foreground/E-motor Start Stop Model/Manual Crank1/Chart1 ==
  state MOTOR_ON
    during: Motor_on=1;
  state MOTOR_OFF
    during: Motor_on=0;
  MOTOR_ON -> MOTOR_OFF [order 2] : [Driving_Mode==2&&Motor_Blend_Factor<0.01]
  MOTOR_ON -> MOTOR_OFF [order 1] : [Driving_Mode==3]
  MOTOR_OFF -> MOTOR_ON [order 1] : [Driving_Mode==1]
  MOTOR_OFF -> MOTOR_ON [order 2] : [Driving_Mode==2&&Motor_Blend_Factor>0.01]
  (default) -> MOTOR_OFF
  data: Driving_Mode input double; Motor_Blend_Factor input double; Motor_on output double

== matlab function Foreground/Stepper Motor/MATLAB Function ==
  data: u input double; y output double; v input double
function y= fcn(u,v)
%#codegen
Diff=u-v;
if abs(Diff)>1
    if Diff>0
        y=1;
    else y=0;
    end
else y=-1;
end

== stateflow chart Foreground/Engine Start Stop Model/Manual Crank/Chart1 ==
  state CRANK_ON
    during: Manual_crank=1;
  state CRANKOFF
    during: Manual_crank=0;
  CRANK_ON -> CRANKOFF : [Driving_Mode==1||Driving_Mode==2]
  CRANKOFF -> CRANK_ON : [Crank_Switch==1&&Driving_Mode==3]
  (default) -> CRANKOFF
  data: Driving_Mode input double; Crank_Switch input double; Manual_crank output double

== stateflow chart Foreground/Engine Start Stop Model/Auto Crank/Chart2 ==
  state CRANK_ON
    during: Automatic_crank=1;
  state CRANKOFF
    during: Automatic_crank=0;
  CRANK_ON -> CRANKOFF [order 1] : [Driving_Mode==1||Driving_Mode==3]
  CRANK_ON -> CRANKOFF [order 2] : [Driving_Mode==2&&Engine_Blend_Factor<0.01]
  CRANKOFF -> CRANK_ON : [Driving_Mode==2&&Engine_Blend_Factor>0.01&&Engine_State==1]
  (default) -> CRANKOFF
  data: Driving_Mode input double; Engine_Blend_Factor input double; Automatic_crank output double; Engine_State input double

== stateflow chart Foreground/Engine Start Stop Model/Manual Crank1/Chart1 ==
  state KILL_ON
    during: Engine_Kill=1;
  state KILL_OFF
    during: Engine_Kill=0;
  KILL_ON -> KILL_OFF [order 2] : [Driving_Mode==2&&Engine_Blend_Factor>0.01]
  KILL_ON -> KILL_OFF [order 1] : [Driving_Mode==3]
  KILL_OFF -> KILL_ON [order 1] : [Driving_Mode==1]
  KILL_OFF -> KILL_ON [order 2] : [Driving_Mode==2&&Engine_Blend_Factor<0.01]
  (default) -> KILL_OFF
  data: Driving_Mode input double; Engine_Blend_Factor input double; Engine_Kill output double

== stateflow chart Foreground/Stepper Motor/Chart ==
  state CW
    state step3
      during:
      Coil1=1;
      Coil2=0;
      Coil3=0;
      Coil4=1;
    state step1
      during:
      Coil1=1;
      Coil2=0;
      Coil3=1;
      Coil4=0;
    state step2
      during:
      Coil1=1;
      Coil2=0;
      Coil3=0;
      Coil4=0;
    state step6
      during:
      Coil1=0;
      Coil2=1;
      Coil3=0;
      Coil4=0;
    state step5
      during:
      Coil1=0;
      Coil2=1;
      Coil3=0;
      Coil4=1;
    state step4
      during:
      Coil1=0;
      Coil2=0;
      Coil3=0;
      Coil4=1;
    state step8
      during:
      Coil1=0;
      Coil2=0;
      Coil3=1;
      Coil4=0;
    state step7
      during:
      Coil1=0;
      Coil2=1;
      Coil3=1;
      Coil4=0;
    (default) -> CW.step1
    CW.step2 -> CW.step3 [order 2] : [step>2]
    CW.step1 -> CW.step2 : [step>1]
    CW.step3 -> CW.step2 [order 1] : [step<3]
    CW.step2 -> CW.step1 [order 1] : [step<2]
    CW.step3 -> CW.step4 [order 2] : [step>3]
    CW.step4 -> CW.step3 [order 1] : [step<4]
    CW.step4 -> CW.step5 [order 2] : [step>4]
    CW.step5 -> CW.step6 [order 2] : [step>5]
    CW.step6 -> CW.step5 [order 1] : [step<6]
    CW.step5 -> CW.step4 [order 1] : [step<5]
    CW.step6 -> CW.step7 [order 2] : [step>6]
    CW.step7 -> CW.step6 [order 1] : [step<7]
    CW.step7 -> CW.step8 [order 2] : [step>7]
    CW.step8 -> CW.step7 : [step<8]
  state CCW
    state step3
      during:
      Coil1=0;
      Coil2=1;
      Coil3=1;
      Coil4=0;
    state step1
      during:
      Coil1=1;
      Coil2=0;
      Coil3=1;
      Coil4=0;
    state step2
      during:
      Coil1=0;
      Coil2=0;
      Coil3=1;
      Coil4=0;
    state step6
      during:
      Coil1=0;
      Coil2=0;
      Coil3=0;
      Coil4=1;
    state step5
      during:
      Coil1=0;
      Coil2=1;
      Coil3=0;
      Coil4=1;
    state step4
      during:
      Coil1=0;
      Coil2=1;
      Coil3=0;
      Coil4=0;
    state step7
      during:
      Coil1=1;
      Coil2=0;
      Coil3=0;
      Coil4=1;
    state step8
      during:
      Coil1=1;
      Coil2=0;
      Coil3=0;
      Coil4=0;
    (default) -> CCW.step1
    CCW.step1 -> CCW.step2 : [step>1]
    CCW.step2 -> CCW.step3 [order 2] : [step>2]
    CCW.step3 -> CCW.step2 [order 1] : [step<3]
    CCW.step2 -> CCW.step1 [order 1] : [step<2]
    CCW.step3 -> CCW.step4 [order 2] : [step>3]
    CCW.step4 -> CCW.step3 [order 1] : [step<4]
    CCW.step5 -> CCW.step6 [order 2] : [step>5]
    CCW.step4 -> CCW.step5 [order 2] : [step>4]
    CCW.step6 -> CCW.step5 [order 1] : [step<6]
    CCW.step5 -> CCW.step4 [order 1] : [step<5]
    CCW.step6 -> CCW.step7 [order 2] : [step>6]
    CCW.step7 -> CCW.step6 [order 1] : [step<7]
    CCW.step7 -> CCW.step8 [order 2] : [step>7]
    CCW.step8 -> CCW.step7 : [step<8]
  state DIR_1
    during:
    Coil1=0
    Coil2=0
    Coil3=0
    Coil4=0
  (junction 196) -> CW [order 2] : [Direction==1]
  (junction 196) -> CCW [order 1] : [Direction==0]
  CW -> (junction 196) [order 2] : [Direction~=1]
  CCW -> (junction 196) [order 2] : [Direction~=1]
  DIR_1 -> (junction 196) : [Direction~=-1]
  CCW -> DIR_1 [order 1] : [Direction==-1]
  CW -> DIR_1 [order 1] : [Direction==-1]
  (default) -> DIR_1
  data: Direction input double; Coil1 output double; Coil2 output double; Coil3 output double; Coil4 output double; step input double
